simulink model "miz_test"  (R2017b)
settings: Solver=VariableStepAuto  StartTime=0.0  StopTime=10.0  RelTol=1e-3
libraries: dspsnks4 x2, commutil2 x2, commdigbbndpm3 x2, commdigbbndam3 x2, commchan3 x1, dspsrcs4 x1, commsink2 x1, dspvision x1
settings Model: Creator=root  LastModifiedBy=root

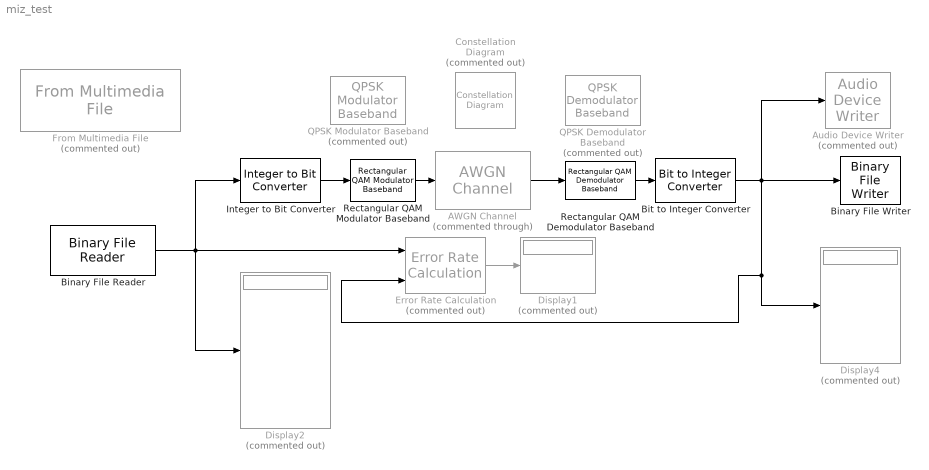
== system miz_test ==
  AWGN Channel : commchan3/AWGN Channel  Commented=through  InputProcessing=Columns as channels (frame based)  seed=67  noiseMode="Signal to noise ratio  (Eb/No)"  EbNodB=60  EsNodB=10  SNRdB=10  bitsPerSym=1  Ps=1  Tsym=1  variance=1
  Audio Device Writer : dspsnks4/Audio Device Writer  Commented=on  Driver=ALSA  Device=Default  InheritSampleRate=off  SampleRate=44100  BitDepth=16-bit integer  BufferSize=4096  NumBuffers=10  DefaultOutputChannelMapping=on  OutputChannelMapping=1:2  OutputNumUnderrunSamples=off  DriverIdx=8  DeviceWarnFlag=''
  Binary File Reader : dspsrcs4/Binary File Reader  Filename=/home/udsdrew/simulink-diagrams-testing/ex.bin  HeaderStructure=struct([])  DataType=int16  SamplesPerFrame=1024  IsDataComplex=off  NumChannels=1  OutputEOF=off  SampleTime=100  SimulateUsing=Code generation
      settings: SourceProductName=DSP System Toolbox  SourceProductBaseCode=DS
  Binary File Writer : dspsnks4/Binary File Writer  Filename=Received.bin  HeaderStructure=struct([])  SimulateUsing=Code generation
      settings: SourceProductName=DSP System Toolbox  SourceProductBaseCode=DS
  Bit to Integer Converter : commutil2/Bit to Integer Converter  nbits=16  bitOrder=MSB first  signedOutputValues=Signed  outDtype=Inherit via internal rule  outDtypeSigned=Inherit via internal rule
  Constellation Diagram : ConstellationDiagram  Commented=on
  Display1 : Display  Commented=on
  Display2 : Display  Commented=on
  Display4 : Display  Commented=on
  Error Rate Calculation : commsink2/Error Rate Calculation  Commented=on  N=0  st_delay=0  cp_mode=Entire frame  subframe=[]  PMode=Port  WsName=ErrorVec  RsMode2=off  stop=off  numErr=100  maxBits=1e6
  From Multimedia File : dspvision/From Multimedia File  Commented=on  inputFilename=C:\Users\bstac\Desktop\Research\Senior Design\04_Let_Me_Be_Myself_mono.wav  loop=on  numPlays=inf  outputStreams=Audio only  videoDataType=single  audioDataType=int16  inheritSampleTime=on  userDefinedSampleTime=1/30  noAudioOutput=off  isIntensityVideo=off  fourcc=RGB  colorVideoFormat=One multidimensional signal  outputEOF=off  dataOrg=Column-major  audioFrameSize=8192  computeAudioFrameSize=off  outSamplingMode=Sample based
      settings: SourceProductBaseCode=VP
  Integer to Bit Converter : commutil2/Integer to Bit Converter  nbits=16  signedInputValues=Signed  bitOrder=MSB first  outDtype=Inherit via internal rule
  QPSK Demodulator Baseband : commdigbbndpm3/QPSK Demodulator Baseband  Commented=on  OutType=Bit  DecType=Hard decision  VarSource=Dialog  Variance=1  Dec=Gray  Ph=pi/4  outDtype1=Inherit via internal rule  outDtype2=int16  derotateFactorWordLen=16  derotateFactorDataTypeStr=Inherit: Same word length as input  derotateFactorLastDataTypeStr=Inherit: Same word length as input
  QPSK Modulator Baseband : commdigbbndpm3/QPSK Modulator Baseband  Commented=on  InType=Integer  Enc=Gray  Ph=pi/4  outDtype=double  outWordLen=16  outUDDataType=sfix(16)  outFracLenMode=Best precision  outFracLen=15  outDataTypeStr=double  outLastDataTypeStr=double
  Rectangular QAM Demodulator Baseband : commdigbbndam3/Rectangular QAM Demodulator Baseband  M=16  OutType=Bit  DecType=Hard decision  VarSource=Dialog  Variance=1  Dec=Binary  Mapping=[0:15]  PowType=Min. distance between symbols  MinDist=1  AvgPow=1  PeakPow=1  Ph=0  outDtype1=Inherit via internal rule  outDtype2=Inherit via internal rule  derotateFactorWordLen=16  derotateFactorDataTypeStr=Inherit: Same word length as input  derotateFactorLastDataTypeStr=Inherit: Same word length as input  denormFactorWordLen=16  denormFactorDataTypeStr=Inherit: Same word length as input  denormFactorLastDataTypeStr=Inherit: Same word length as input  prodOutWordLen=32  prodOutOverflowMode=Wrap  prodOutRoundingMode=Floor  prodOutOvFlMode=off  prodOutOvFlModeLastStrValue=off  sumWordLen=32
  Rectangular QAM Modulator Baseband : commdigbbndam3/Rectangular QAM Modulator Baseband  M=16  InType=Bit  Enc=Binary  Mapping=[0:15]  PowType=Min. distance between symbols  MinDist=2  AvgPow=1  PeakPow=1  Ph=0  outDtype=Inherit via back propagation  outWordLen=16  outUDDataType=sfix(16)  outFracLenMode=Best precision  outFracLen=15  outDataTypeStr=Inherit: Inherit via back propagation  outLastDataTypeStr=Inherit: Inherit via back propagation
  wires:
  Error Rate Calculation/1 -> Display1/1
  Bit to Integer Converter/1 -> Binary File Writer/1, Audio Device Writer/1, Display4/1, Error Rate Calculation/2
  Binary File Reader/1 -> Error Rate Calculation/1, Integer to Bit Converter/1, Display2/1
  Rectangular QAM Modulator Baseband/1 -> AWGN Channel/1
  Integer to Bit Converter/1 -> Rectangular QAM Modulator Baseband/1
  Rectangular QAM Demodulator Baseband/1 -> Bit to Integer Converter/1
  AWGN Channel/1 -> Rectangular QAM Demodulator Baseband/1
